simulink model "HW8_2"  (R2020b)
settings: Solver=FixedStepAuto  StartTime=0.0  StopTime=10  RelTol=1e-3
settings Model: Creator=ricky  LastModifiedBy=ricky

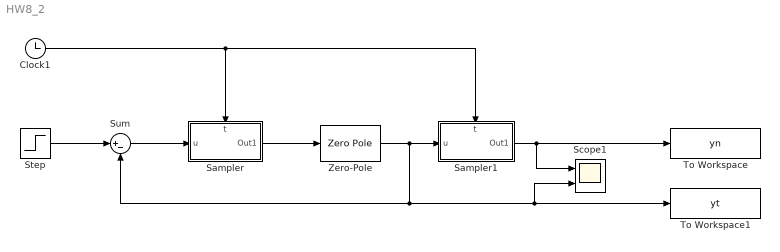
== system HW8_2 ==
  Clock1 : Clock
  Sampler : Subsystem
      settings: PortSchema="{\"entries\":[{\"content\":{\"sides\":[{\"content\":{\"connectorIds\":[\"In1\"]},\"type\":\"ConnectorPlacement.EquallySpacedRectSide\",\"uuid\":\"3b193190-d7b9-4088-bdd7-347e859ba189\"},{\"content\":{\"connectorIds\":[\"Out1\"],\"side\":\"RIGHT\"},\"type\":\"ConnectorPlacement.EquallySpacedRectSide\",\"uuid\":\"29255df0-e00c-48af-be35-0f1e8e26bd75\"},{\"content\":{\"connectorIds\":[\"In2\"],\"side\":\"TOP\"},\"type\":\"ConnectorPlacement.EquallySpacedRectSide\",\"uuid\":\"cd4a92b5-2c2f-41a5-bdb6-e490de70a208\"},{\"content\":{\"connectorIds\":[],\"side\":\"HIDDEN\"},\"type\":\"ConnectorPlacement.EquallySpacedRectSide\",\"uuid\":\"e5436d80-6dbc-4975-807b-5570bf36fe7d\"}]},\"type\":\"ConnectorPlacement.EquallySpacedConnector\",\"uuid\":\"2a3ee3c5-b217-48f6-b138-b512f102837a\"}],\"packageUris\":[\"http://schema.mathworks.com/mf0/Connector/R2020b\"],\"version\":\"1.0\"}"
      mask Display: image('$imagefile'); % Use "Edit Image" on toolstrip to change.
  Sampler1 : Subsystem
      settings: PortSchema="{\"entries\":[{\"content\":{\"sides\":[{\"content\":{\"connectorIds\":[\"In1\"]},\"type\":\"ConnectorPlacement.EquallySpacedRectSide\",\"uuid\":\"3b193190-d7b9-4088-bdd7-347e859ba189\"},{\"content\":{\"connectorIds\":[\"Out1\"],\"side\":\"RIGHT\"},\"type\":\"ConnectorPlacement.EquallySpacedRectSide\",\"uuid\":\"29255df0-e00c-48af-be35-0f1e8e26bd75\"},{\"content\":{\"connectorIds\":[\"In2\"],\"side\":\"TOP\"},\"type\":\"ConnectorPlacement.EquallySpacedRectSide\",\"uuid\":\"cd4a92b5-2c2f-41a5-bdb6-e490de70a208\"},{\"content\":{\"connectorIds\":[],\"side\":\"HIDDEN\"},\"type\":\"ConnectorPlacement.EquallySpacedRectSide\",\"uuid\":\"e5436d80-6dbc-4975-807b-5570bf36fe7d\"}]},\"type\":\"ConnectorPlacement.EquallySpacedConnector\",\"uuid\":\"2a3ee3c5-b217-48f6-b138-b512f102837a\"}],\"packageUris\":[\"http://schema.mathworks.com/mf0/Connector/R2020b\"],\"version\":\"1.0\"}"
      mask Display: image('$imagefile'); % Use "Edit Image" on toolstrip to change.
  Scope1 : Scope  NumInputPorts=2
  Step : Step  Time=0  SampleTime=0
  Sum : Sum  Inputs=|+-
  To Workspace : ToWorkspace  VariableName=yn  SaveFormat=Timeseries  SampleTime=-1
  To Workspace1 : ToWorkspace  VariableName=yt  SaveFormat=Timeseries  SampleTime=-1
  Zero-Pole : ZeroPole  Zeros=[]  Poles=[0 -1]
  wires:
  Clock1/1 -> Sampler1/2(t), Sampler/2(t)
  Sampler/1(Out1) -> Zero-Pole/1
  Zero-Pole/1 -> Sum/2, To Workspace1/1, Scope1/2, Sampler1/1(u)
  Sampler1/1(Out1) -> To Workspace/1, Scope1/1
  Step/1 -> Sum/1
  Sum/1 -> Sampler/1(u)

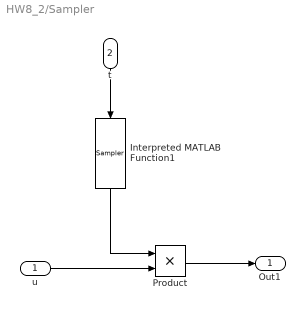
== system HW8_2/Sampler ==
  u : Inport
  t : Inport  Port=2
  Interpreted MATLAB Function1 : MATLABFcn  MATLABFcn=Sampler
  Product : Product
  Out1 : Outport
  wires:
  u/1 -> Product/2
  Interpreted MATLAB Function1/1 -> Product/1
  Product/1 -> Out1/1
  t/1 -> Interpreted MATLAB Function1/1

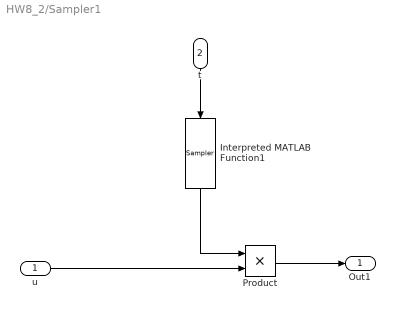
== system HW8_2/Sampler1 ==
  u : Inport
  t : Inport  Port=2
  Interpreted MATLAB Function1 : MATLABFcn  MATLABFcn=Sampler
  Product : Product
  Out1 : Outport
  wires:
  u/1 -> Product/2
  Interpreted MATLAB Function1/1 -> Product/1
  Product/1 -> Out1/1
  t/1 -> Interpreted MATLAB Function1/1
